simulink model "dsss"  (Simulink 7.1)
settings: Solver=ode45  StartTime=0.0  StopTime=0.80  RelTol=1e-3
libraries: simulink x264, dspbuff3 x24, dspxfrm3 x8, commsynccomp2 x5, dspsigops x4, dspobslib x4, dsparch4 x3, commutil2 x2, commseqgen2 x1, commfilt2 x1, commsink2 x1, dspspect3 x1
(part 2 of 4)

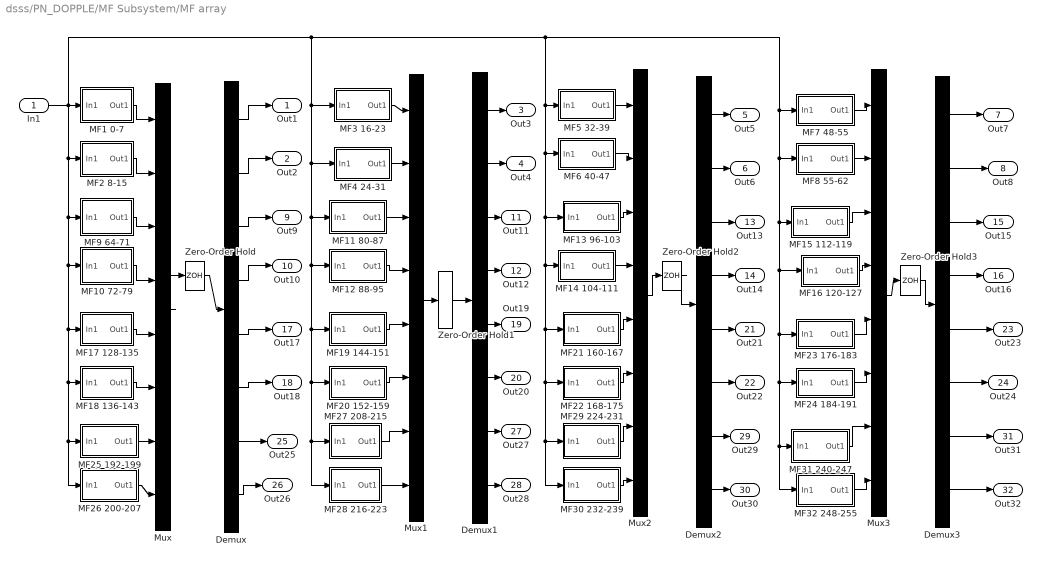
== system dsss/PN_DOPPLE/MF Subsystem/MF array ==
  In1 : Inport  OutDataType=sfix(16)  OutScaling=2^0
  Demux{,1..3} (4 alike) : Demux  Outputs=8
  MF1 0-7 : Subsystem
  MF10 72-79 : Subsystem
  MF11 80-87 : Subsystem
  MF12 88-95 : Subsystem
  MF13 96-103 : Subsystem
  MF14 104-111 : Subsystem
  MF15 112-119 : Subsystem
  MF16 120-127 : Subsystem
  MF17 128-135 : Subsystem
  MF18 136-143 : Subsystem
  MF19 144-151 : Subsystem
  MF2 8-15 : Subsystem
  MF20 152-159 : Subsystem
  MF21 160-167 : Subsystem
  MF22 168-175 : Subsystem
  MF23 176-183 : Subsystem
  MF24 184-191 : Subsystem
  MF25 192-199 : Subsystem
  MF26 200-207 : Subsystem
  MF27 208-215 : Subsystem
  MF28 216-223 : Subsystem
  MF29 224-231 : Subsystem
  MF3 16-23 : Subsystem
  MF30 232-239 : Subsystem
  MF31 240-247 : Subsystem
  MF32 248-255 : Subsystem
  MF4 24-31 : Subsystem
  MF5 32-39 : Subsystem
  MF6 40-47 : Subsystem
  MF7 48-55 : Subsystem
  MF8 55-62 : Subsystem
  MF9 64-71 : Subsystem
  Mux{,1..3} (4 alike) : Mux  Inputs=8
  Zero-Order Hold{,1..3} (4 alike) : ZeroOrderHold  SampleTime=1/255000
  Out1 : Outport  OutDataType=sfix(16)  OutScaling=2^0
  Out2 : Outport  Port=2  OutDataType=sfix(16)  OutScaling=2^0
  Out3 : Outport  Port=3  OutDataType=sfix(16)  OutScaling=2^0
  Out4 : Outport  Port=4  OutDataType=sfix(16)  OutScaling=2^0
  Out5 : Outport  Port=5  OutDataType=sfix(16)  OutScaling=2^0
  Out6 : Outport  Port=6  OutDataType=sfix(16)  OutScaling=2^0
  Out7 : Outport  Port=7  OutDataType=sfix(16)  OutScaling=2^0
  Out8 : Outport  Port=8  OutDataType=sfix(16)  OutScaling=2^0
  Out9 : Outport  Port=9  OutDataType=sfix(16)  OutScaling=2^0
  Out10 : Outport  Port=10  OutDataType=sfix(16)  OutScaling=2^0
  Out11 : Outport  Port=11  OutDataType=sfix(16)  OutScaling=2^0
  Out12 : Outport  Port=12  OutDataType=sfix(16)  OutScaling=2^0
  Out13 : Outport  Port=13  OutDataType=sfix(16)  OutScaling=2^0
  Out14 : Outport  Port=14  OutDataType=sfix(16)  OutScaling=2^0
  Out15 : Outport  Port=15  OutDataType=sfix(16)  OutScaling=2^0
  Out16 : Outport  Port=16  OutDataType=sfix(16)  OutScaling=2^0
  Out17 : Outport  Port=17  OutDataType=sfix(16)  OutScaling=2^0
  Out18 : Outport  Port=18  OutDataType=sfix(16)  OutScaling=2^0
  Out19 : Outport  Port=19  OutDataType=sfix(16)  OutScaling=2^0
  Out20 : Outport  Port=20  OutDataType=sfix(16)  OutScaling=2^0
  Out21 : Outport  Port=21  OutDataType=sfix(16)  OutScaling=2^0
  Out22 : Outport  Port=22  OutDataType=sfix(16)  OutScaling=2^0
  Out23 : Outport  Port=23  OutDataType=sfix(16)  OutScaling=2^0
  Out24 : Outport  Port=24  OutDataType=sfix(16)  OutScaling=2^0
  Out25 : Outport  Port=25  OutDataType=sfix(16)  OutScaling=2^0
  Out26 : Outport  Port=26  OutDataType=sfix(16)  OutScaling=2^0
  Out27 : Outport  Port=27  OutDataType=sfix(16)  OutScaling=2^0
  Out28 : Outport  Port=28  OutDataType=sfix(16)  OutScaling=2^0
  Out29 : Outport  Port=29  OutDataType=sfix(16)  OutScaling=2^0
  Out30 : Outport  Port=30  OutDataType=sfix(16)  OutScaling=2^0
  Out31 : Outport  Port=31  OutDataType=sfix(16)  OutScaling=2^0
  Out32 : Outport  Port=32  OutDataType=sfix(16)  OutScaling=2^0
  wires:
  Zero-Order Hold3/1 -> Demux3/1
  Mux3/1 -> Zero-Order Hold3/1
  Zero-Order Hold2/1 -> Demux2/1
  Mux2/1 -> Zero-Order Hold2/1
  Zero-Order Hold1/1 -> Demux1/1
  Mux1/1 -> Zero-Order Hold1/1
  Zero-Order Hold/1 -> Demux/1
  Mux/1 -> Zero-Order Hold/1
  In1/1 -> MF1 0-7/1(In1), MF3 16-23/1(In1), MF11 80-87/1(In1), MF19 144-151/1(In1), MF20 152-159/1(In1), MF27 208-215/1(In1), MF28 216-223/1(In1), MF12 88-95/1(In1), MF4 24-31/1(In1), MF5 32-39/1(In1), MF13 96-103/1(In1), MF21 160-167/1(In1), MF22 168-175/1(In1), MF29 224-231/1(In1), MF30 232-239/1(In1), MF14 104-111/1(In1), MF6 40-47/1(In1), MF7 48-55/1(In1), MF23 176-183/1(In1), MF24 184-191/1(In1), MF31 240-247/1(In1), MF32 248-255/1(In1), MF16 120-127/1(In1), MF15 112-119/1(In1), MF8 55-62/1(In1), MF9 64-71/1(In1), MF17 128-135/1(In1), MF18 136-143/1(In1), MF25 192-199/1(In1), MF26 200-207/1(In1), MF10 72-79/1(In1), MF2 8-15/1(In1)
  MF1 0-7/1(Out1) -> Mux/1
  MF2 8-15/1(Out1) -> Mux/2
  MF9 64-71/1(Out1) -> Mux/3
  MF10 72-79/1(Out1) -> Mux/4
  MF17 128-135/1(Out1) -> Mux/5
  MF18 136-143/1(Out1) -> Mux/6
  MF25 192-199/1(Out1) -> Mux/7
  MF26 200-207/1(Out1) -> Mux/8
  Demux/1 -> Out1/1
  Demux/2 -> Out2/1
  Demux/3 -> Out9/1
  Demux/4 -> Out10/1
  Demux/5 -> Out17/1
  Demux/6 -> Out18/1
  Demux/7 -> Out25/1
  Demux/8 -> Out26/1
  MF3 16-23/1(Out1) -> Mux1/1
  MF4 24-31/1(Out1) -> Mux1/2
  MF11 80-87/1(Out1) -> Mux1/3
  MF12 88-95/1(Out1) -> Mux1/4
  MF19 144-151/1(Out1) -> Mux1/5
  MF20 152-159/1(Out1) -> Mux1/6
  MF27 208-215/1(Out1) -> Mux1/7
  MF28 216-223/1(Out1) -> Mux1/8
  Demux1/1 -> Out3/1
  Demux1/2 -> Out4/1
  Demux1/3 -> Out11/1
  Demux1/4 -> Out12/1
  Demux1/5 -> Out19/1
  Demux1/6 -> Out20/1
  Demux1/7 -> Out27/1
  Demux1/8 -> Out28/1
  MF5 32-39/1(Out1) -> Mux2/1
  MF6 40-47/1(Out1) -> Mux2/2
  MF13 96-103/1(Out1) -> Mux2/3
  MF14 104-111/1(Out1) -> Mux2/4
  MF21 160-167/1(Out1) -> Mux2/5
  MF22 168-175/1(Out1) -> Mux2/6
  MF29 224-231/1(Out1) -> Mux2/7
  MF30 232-239/1(Out1) -> Mux2/8
  Demux2/1 -> Out5/1
  Demux2/2 -> Out6/1
  Demux2/3 -> Out13/1
  Demux2/4 -> Out14/1
  Demux2/5 -> Out21/1
  Demux2/6 -> Out22/1
  Demux2/7 -> Out29/1
  Demux2/8 -> Out30/1
  MF7 48-55/1(Out1) -> Mux3/1
  MF8 55-62/1(Out1) -> Mux3/2
  MF15 112-119/1(Out1) -> Mux3/3
  MF16 120-127/1(Out1) -> Mux3/4
  MF23 176-183/1(Out1) -> Mux3/5
  MF24 184-191/1(Out1) -> Mux3/6
  MF31 240-247/1(Out1) -> Mux3/7
  MF32 248-255/1(Out1) -> Mux3/8
  Demux3/1 -> Out7/1
  Demux3/2 -> Out8/1
  Demux3/3 -> Out15/1
  Demux3/4 -> Out16/1
  Demux3/5 -> Out23/1
  Demux3/6 -> Out24/1
  Demux3/7 -> Out31/1
  Demux3/8 -> Out32/1

== system dsss/PN_DOPPLE/FFT compensate/Subsystem/Subsystem ==
  In1 : Inport  OutDataType=sfix(16)  OutScaling=2^0
  Constant : Constant  OutDataType=sfix(16)  OutScaling=2^0
  Constant1 : Constant  Value=0  OutDataType=sfix(16)  OutScaling=2^0
  Constant2 : Constant  Value=0  OutDataType=sfix(16)  OutScaling=2^0
  Product : Product  OutDataType=sfix(16)  OutScaling=2^0  RndMeth=Zero
  Switch : Switch  Threshold=65
  Out1 : Outport  OutDataType=sfix(16)  OutScaling=2^0
  wires:
  Constant/1 -> Switch/1
  Constant1/1 -> Switch/3
  Switch/1 -> Product/1
  Constant2/1 -> Product/2
  In1/1 -> Switch/2
  Product/1 -> Out1/1

== system dsss/PN_DOPPLE/FFT compensate/Subsystem/Subsystem1 ==
  In1 : Inport  OutDataType=sfix(16)  OutScaling=2^0
  Constant : Constant  OutDataType=sfix(16)  OutScaling=2^0
  Constant1 : Constant  Value=0  OutDataType=sfix(16)  OutScaling=2^0
  Constant2 : Constant  Value=10  OutDataType=sfix(16)  OutScaling=2^0
  Product : Product  OutDataType=sfix(16)  OutScaling=2^0  RndMeth=Zero
  Switch : Switch  Threshold=65
  Out1 : Outport  OutDataType=sfix(16)  OutScaling=2^0
  wires:
  Product/1 -> Out1/1
  In1/1 -> Switch/2
  Constant2/1 -> Product/2
  Switch/1 -> Product/1
  Constant1/1 -> Switch/3
  Constant/1 -> Switch/1

== system dsss/PN_DOPPLE/FFT compensate/Subsystem/Subsystem10 ==
  In1 : Inport  OutDataType=sfix(16)  OutScaling=2^0
  Constant : Constant  OutDataType=sfix(16)  OutScaling=2^0
  Constant1 : Constant  Value=0  OutDataType=sfix(16)  OutScaling=2^0
  Constant2 : Constant  Value=100  OutDataType=sfix(16)  OutScaling=2^0
  Product : Product  OutDataType=sfix(16)  OutScaling=2^0  RndMeth=Zero
  Switch : Switch  Threshold=65
  Out1 : Outport  OutDataType=sfix(16)  OutScaling=2^0
  wires:
  Constant/1 -> Switch/1
  Constant1/1 -> Switch/3
  Switch/1 -> Product/1
  Constant2/1 -> Product/2
  In1/1 -> Switch/2
  Product/1 -> Out1/1

== system dsss/PN_DOPPLE/FFT compensate/Subsystem/Subsystem11 ==
  In1 : Inport  OutDataType=sfix(16)  OutScaling=2^0
  Constant : Constant  OutDataType=sfix(16)  OutScaling=2^0
  Constant1 : Constant  Value=0  OutDataType=sfix(16)  OutScaling=2^0
  Constant2 : Constant  Value=110  OutDataType=sfix(16)  OutScaling=2^0
  Product : Product  OutDataType=sfix(16)  OutScaling=2^0  RndMeth=Zero
  Switch : Switch  Threshold=65
  Out1 : Outport  OutDataType=sfix(16)  OutScaling=2^0
  wires:
  Product/1 -> Out1/1
  In1/1 -> Switch/2
  Constant2/1 -> Product/2
  Switch/1 -> Product/1
  Constant1/1 -> Switch/3
  Constant/1 -> Switch/1

== system dsss/PN_DOPPLE/FFT compensate/Subsystem/Subsystem12 ==
  In1 : Inport  OutDataType=sfix(16)  OutScaling=2^0
  Constant : Constant  OutDataType=sfix(16)  OutScaling=2^0
  Constant1 : Constant  Value=0  OutDataType=sfix(16)  OutScaling=2^0
  Constant2 : Constant  Value=120  OutDataType=sfix(16)  OutScaling=2^0
  Product : Product  OutDataType=sfix(16)  OutScaling=2^0  RndMeth=Zero
  Switch : Switch  Threshold=65
  Out1 : Outport  OutDataType=sfix(16)  OutScaling=2^0
  wires:
  Constant/1 -> Switch/1
  Constant1/1 -> Switch/3
  Switch/1 -> Product/1
  Constant2/1 -> Product/2
  In1/1 -> Switch/2
  Product/1 -> Out1/1

== system dsss/PN_DOPPLE/FFT compensate/Subsystem/Subsystem13 ==
  In1 : Inport  OutDataType=sfix(16)  OutScaling=2^0
  Constant : Constant  OutDataType=sfix(16)  OutScaling=2^0
  Constant1 : Constant  Value=0  OutDataType=sfix(16)  OutScaling=2^0
  Constant2 : Constant  Value=130  OutDataType=sfix(16)  OutScaling=2^0
  Product : Product  OutDataType=sfix(16)  OutScaling=2^0  RndMeth=Zero
  Switch : Switch  Threshold=65
  Out1 : Outport  OutDataType=sfix(16)  OutScaling=2^0
  wires:
  Product/1 -> Out1/1
  In1/1 -> Switch/2
  Constant2/1 -> Product/2
  Switch/1 -> Product/1
  Constant1/1 -> Switch/3
  Constant/1 -> Switch/1

== system dsss/PN_DOPPLE/FFT compensate/Subsystem/Subsystem14 ==
  In1 : Inport  OutDataType=sfix(16)  OutScaling=2^0
  Constant : Constant  OutDataType=sfix(16)  OutScaling=2^0
  Constant1 : Constant  Value=0  OutDataType=sfix(16)  OutScaling=2^0
  Constant2 : Constant  Value=140  OutDataType=sfix(16)  OutScaling=2^0
  Product : Product  OutDataType=sfix(16)  OutScaling=2^0  RndMeth=Zero
  Switch : Switch  Threshold=65
  Out1 : Outport  OutDataType=sfix(16)  OutScaling=2^0
  wires:
  Constant/1 -> Switch/1
  Constant1/1 -> Switch/3
  Switch/1 -> Product/1
  Constant2/1 -> Product/2
  In1/1 -> Switch/2
  Product/1 -> Out1/1

== system dsss/PN_DOPPLE/FFT compensate/Subsystem/Subsystem15 ==
  In1 : Inport  OutDataType=sfix(16)  OutScaling=2^0
  Constant : Constant  OutDataType=sfix(16)  OutScaling=2^0
  Constant1 : Constant  Value=0  OutDataType=sfix(16)  OutScaling=2^0
  Constant2 : Constant  Value=150  OutDataType=sfix(16)  OutScaling=2^0
  Product : Product  OutDataType=sfix(16)  OutScaling=2^0  RndMeth=Zero
  Switch : Switch  Threshold=65
  Out1 : Outport  OutDataType=sfix(16)  OutScaling=2^0
  wires:
  Product/1 -> Out1/1
  In1/1 -> Switch/2
  Constant2/1 -> Product/2
  Switch/1 -> Product/1
  Constant1/1 -> Switch/3
  Constant/1 -> Switch/1

== system dsss/PN_DOPPLE/FFT compensate/Subsystem/Subsystem2 ==
  In1 : Inport  OutDataType=sfix(16)  OutScaling=2^0
  Constant : Constant  OutDataType=sfix(16)  OutScaling=2^0
  Constant1 : Constant  Value=0  OutDataType=sfix(16)  OutScaling=2^0
  Constant2 : Constant  Value=20  OutDataType=sfix(16)  OutScaling=2^0
  Product : Product  OutDataType=sfix(16)  OutScaling=2^0  RndMeth=Zero
  Switch : Switch  Threshold=65
  Out1 : Outport  OutDataType=sfix(16)  OutScaling=2^0
  wires:
  Constant/1 -> Switch/1
  Constant1/1 -> Switch/3
  Switch/1 -> Product/1
  Constant2/1 -> Product/2
  In1/1 -> Switch/2
  Product/1 -> Out1/1

== system dsss/PN_DOPPLE/FFT compensate/Subsystem/Subsystem3 ==
  In1 : Inport  OutDataType=sfix(16)  OutScaling=2^0
  Constant : Constant  OutDataType=sfix(16)  OutScaling=2^0
  Constant1 : Constant  Value=0  OutDataType=sfix(16)  OutScaling=2^0
  Constant2 : Constant  Value=30  OutDataType=sfix(16)  OutScaling=2^0
  Product : Product  OutDataType=sfix(16)  OutScaling=2^0  RndMeth=Zero
  Switch : Switch  Threshold=65
  Out1 : Outport  OutDataType=sfix(16)  OutScaling=2^0
  wires:
  Product/1 -> Out1/1
  In1/1 -> Switch/2
  Constant2/1 -> Product/2
  Switch/1 -> Product/1
  Constant1/1 -> Switch/3
  Constant/1 -> Switch/1

== system dsss/PN_DOPPLE/FFT compensate/Subsystem/Subsystem4 ==
  In1 : Inport  OutDataType=sfix(16)  OutScaling=2^0
  Constant : Constant  OutDataType=sfix(16)  OutScaling=2^0
  Constant1 : Constant  Value=0  OutDataType=sfix(16)  OutScaling=2^0
  Constant2 : Constant  Value=40  OutDataType=sfix(16)  OutScaling=2^0
  Product : Product  OutDataType=sfix(16)  OutScaling=2^0  RndMeth=Zero
  Switch : Switch  Threshold=65
  Out1 : Outport  OutDataType=sfix(16)  OutScaling=2^0
  wires:
  Constant/1 -> Switch/1
  Constant1/1 -> Switch/3
  Switch/1 -> Product/1
  Constant2/1 -> Product/2
  In1/1 -> Switch/2
  Product/1 -> Out1/1

== system dsss/PN_DOPPLE/FFT compensate/Subsystem/Subsystem5 ==
  In1 : Inport  OutDataType=sfix(16)  OutScaling=2^0
  Constant : Constant  OutDataType=sfix(16)  OutScaling=2^0
  Constant1 : Constant  Value=0  OutDataType=sfix(16)  OutScaling=2^0
  Constant2 : Constant  Value=50  OutDataType=sfix(16)  OutScaling=2^0
  Product : Product  OutDataType=sfix(16)  OutScaling=2^0  RndMeth=Zero
  Switch : Switch  Threshold=65
  Out1 : Outport  OutDataType=sfix(16)  OutScaling=2^0
  wires:
  Product/1 -> Out1/1
  In1/1 -> Switch/2
  Constant2/1 -> Product/2
  Switch/1 -> Product/1
  Constant1/1 -> Switch/3
  Constant/1 -> Switch/1

== system dsss/PN_DOPPLE/FFT compensate/Subsystem/Subsystem6 ==
  In1 : Inport  OutDataType=sfix(16)  OutScaling=2^0
  Constant : Constant  OutDataType=sfix(16)  OutScaling=2^0
  Constant1 : Constant  Value=0  OutDataType=sfix(16)  OutScaling=2^0
  Constant2 : Constant  Value=60  OutDataType=sfix(16)  OutScaling=2^0
  Product : Product  OutDataType=sfix(16)  OutScaling=2^0  RndMeth=Zero
  Switch : Switch  Threshold=65
  Out1 : Outport  OutDataType=sfix(16)  OutScaling=2^0
  wires:
  Constant/1 -> Switch/1
  Constant1/1 -> Switch/3
  Switch/1 -> Product/1
  Constant2/1 -> Product/2
  In1/1 -> Switch/2
  Product/1 -> Out1/1

== system dsss/PN_DOPPLE/FFT compensate/Subsystem/Subsystem7 ==
  In1 : Inport  OutDataType=sfix(16)  OutScaling=2^0
  Constant : Constant  OutDataType=sfix(16)  OutScaling=2^0
  Constant1 : Constant  Value=0  OutDataType=sfix(16)  OutScaling=2^0
  Constant2 : Constant  Value=70  OutDataType=sfix(16)  OutScaling=2^0
  Product : Product  OutDataType=sfix(16)  OutScaling=2^0  RndMeth=Zero
  Switch : Switch  Threshold=65
  Out1 : Outport  OutDataType=sfix(16)  OutScaling=2^0
  wires:
  Product/1 -> Out1/1
  In1/1 -> Switch/2
  Constant2/1 -> Product/2
  Switch/1 -> Product/1
  Constant1/1 -> Switch/3
  Constant/1 -> Switch/1

== system dsss/PN_DOPPLE/FFT compensate/Subsystem/Subsystem8 ==
  In1 : Inport  OutDataType=sfix(16)  OutScaling=2^0
  Constant : Constant  OutDataType=sfix(16)  OutScaling=2^0
  Constant1 : Constant  Value=0  OutDataType=sfix(16)  OutScaling=2^0
  Constant2 : Constant  Value=80  OutDataType=sfix(16)  OutScaling=2^0
  Product : Product  OutDataType=sfix(16)  OutScaling=2^0  RndMeth=Zero
  Switch : Switch  Threshold=65
  Out1 : Outport  OutDataType=sfix(16)  OutScaling=2^0
  wires:
  Constant/1 -> Switch/1
  Constant1/1 -> Switch/3
  Switch/1 -> Product/1
  Constant2/1 -> Product/2
  In1/1 -> Switch/2
  Product/1 -> Out1/1

== system dsss/PN_DOPPLE/FFT compensate/Subsystem/Subsystem9 ==
  In1 : Inport  OutDataType=sfix(16)  OutScaling=2^0
  Constant : Constant  OutDataType=sfix(16)  OutScaling=2^0
  Constant1 : Constant  Value=0  OutDataType=sfix(16)  OutScaling=2^0
  Constant2 : Constant  Value=90  OutDataType=sfix(16)  OutScaling=2^0
  Product : Product  OutDataType=sfix(16)  OutScaling=2^0  RndMeth=Zero
  Switch : Switch  Threshold=65
  Out1 : Outport  OutDataType=sfix(16)  OutScaling=2^0
  wires:
  Product/1 -> Out1/1
  In1/1 -> Switch/2
  Constant2/1 -> Product/2
  Switch/1 -> Product/1
  Constant1/1 -> Switch/3
  Constant/1 -> Switch/1

== system dsss/PN_DOPPLE/Local PN/local PN sequence Include Track/Clock ==
  In2 : Inport  Orientation=left  OutDataType=sfix(16)  OutScaling=2^0
  Constant : Constant  Orientation=left  OutDataType=sfix(16)  OutScaling=2^0
  Constant1 : Constant  Orientation=left  Value=0  OutDataType=sfix(16)  OutScaling=2^0
  Continuous-Time VCO : commsynccomp2/Continuous-Time VCO  Orientation=left  SystemSampleTime=-1  Ac=1  Fc=255000  Kc=0.15  Ph=-pi/2
  Switch : Switch  Orientation=left
  Out1 : Outport  Orientation=left  OutDataType=sfix(16)  OutScaling=2^0
  wires:
  Constant1/1 -> Switch/3
  Constant/1 -> Switch/1
  Continuous-Time VCO/1 -> Switch/2
  Switch/1 -> Out1/1
  In2/1 -> Continuous-Time VCO/1

== system dsss/PN_DOPPLE/Local PN/local PN sequence Include Track/Local System ==
  In1 : Inport  OutDataType=sfix(16)  OutScaling=2^0
  Data Type Conversion : DataTypeConversion  OutDataTypeMode=double  OutDataType=sfix(16)  OutScaling=2^0  OutDataTypeStr=double
  Zero-Order Hold3 : ZeroOrderHold  SampleTime=1/255e3
  "[1 0 0 1 1 1 0 1]PN" : Subsystem  TreatAsAtomicUnit=on
  "[1 0 0 1 1 1 0 1]" : Outport  OutDataType=sfix(16)  OutScaling=2^0
  wires:
  In1/1 -> "[1 0 0 1 1 1 0 1]PN"/Trigger, "[1 0 0 1 1 1 0 1]PN"/1(In1)
  "[1 0 0 1 1 1 0 1]PN"/1(Out1) -> Data Type Conversion/1
  Zero-Order Hold3/1 -> "[1 0 0 1 1 1 0 1]"/1
  Data Type Conversion/1 -> Zero-Order Hold3/1

== system dsss/PN_DOPPLE/Local PN/logic control/Triggered Subsystem ==
  Trigger : TriggerPort
  Constant : Constant  OutDataType=sfix(16)  OutScaling=2^0
  Logical Operator : Logic  Operator=XOR  AllPortsSameDT=off  OutDataTypeMode=boolean  OutDataTypeStr=boolean
  Scope : Scope
      settings: SaveName=ScopeData2
  Unit Delay : UnitDelay  Orientation=left  SampleTime=-1
  Out2 : Outport  OutDataType=sfix(16)  OutScaling=2^0
  wires:
  Constant/1 -> Logical Operator/1
  Logical Operator/1 -> Scope/1, Out2/1, Unit Delay/1
  Unit Delay/1 -> Logical Operator/2

== system dsss/PN_DOPPLE/Local PN/threshold deside stop and start/Triggered Subsystem ==
  Trigger : TriggerPort
  Constant1 : Constant  OutDataType=sfix(16)  OutScaling=2^0
  Logical Operator : Logic  Operator=XOR  AllPortsSameDT=off  OutDataTypeMode=boolean  OutDataTypeStr=boolean
  Unit Delay : UnitDelay  Orientation=left  SampleTime=-1
  Out1 : Outport  OutDataType=sfix(16)  OutScaling=2^0
  wires:
  Unit Delay/1 -> Logical Operator/2
  Logical Operator/1 -> Out1/1, Unit Delay/1
  Constant1/1 -> Logical Operator/1

== system dsss/PN_DOPPLE/MF Subsystem/MF array/MF1 0-7 ==
  In1 : Inport  OutDataType=sfix(16)  OutScaling=2^0
  Add : Sum  Inputs=++++++++  OutDataType=sfix(16)  OutScaling=2^-10
  Subsystem : Subsystem
  Out1 : Outport  OutDataType=sfix(16)  OutScaling=2^0
  wires:
  Add/1 -> Out1/1
  In1/1 -> Subsystem/1(In1)
  Subsystem/1(Out1) -> Add/1
  Subsystem/2(Out2) -> Add/2
  Subsystem/3(Out3) -> Add/3
  Subsystem/4(Out4) -> Add/4
  Subsystem/5(Out5) -> Add/5
  Subsystem/6(Out6) -> Add/6
  Subsystem/7(Out7) -> Add/7
  Subsystem/8(Out8) -> Add/8

== system dsss/PN_DOPPLE/MF Subsystem/MF array/MF10 72-79 ==
  In1 : Inport  OutDataType=sfix(16)  OutScaling=2^0
  Add : Sum  Inputs=++++++++  OutDataType=sfix(16)  OutScaling=2^-10
  Subsystem : Subsystem
  Out1 : Outport  OutDataType=sfix(16)  OutScaling=2^0
  wires:
  Subsystem/8(Out8) -> Add/8
  Subsystem/7(Out7) -> Add/7
  Subsystem/6(Out6) -> Add/6
  Subsystem/5(Out5) -> Add/5
  Subsystem/4(Out4) -> Add/4
  Subsystem/3(Out3) -> Add/3
  Subsystem/2(Out2) -> Add/2
  Subsystem/1(Out1) -> Add/1
  In1/1 -> Subsystem/1(In1)
  Add/1 -> Out1/1

== system dsss/PN_DOPPLE/MF Subsystem/MF array/MF11 80-87 ==
  In1 : Inport  OutDataType=sfix(16)  OutScaling=2^0
  Add : Sum  Inputs=++++++++  OutDataType=sfix(16)  OutScaling=2^-10
  Subsystem : Subsystem
  Out1 : Outport  OutDataType=sfix(16)  OutScaling=2^0
  wires:
  In1/1 -> Subsystem/1(In1)
  Add/1 -> Out1/1
  Subsystem/1(Out3) -> Add/1
  Subsystem/2(Out4) -> Add/2
  Subsystem/3(Out7) -> Add/3
  Subsystem/4(Out8) -> Add/4
  Subsystem/5(Out9) -> Add/5
  Subsystem/6(Out11) -> Add/6
  Subsystem/7(Out14) -> Add/7
  Subsystem/8(Out15) -> Add/8

== system dsss/PN_DOPPLE/MF Subsystem/MF array/MF12 88-95 ==
  In1 : Inport  OutDataType=sfix(16)  OutScaling=2^0
  Add : Sum  Inputs=++++++++  OutDataType=sfix(16)  OutScaling=2^-10
  Subsystem : Subsystem
  Out1 : Outport  OutDataType=sfix(16)  OutScaling=2^0
  wires:
  Add/1 -> Out1/1
  In1/1 -> Subsystem/1(In1)
  Subsystem/1(Out1) -> Add/1
  Subsystem/2(Out5) -> Add/2
  Subsystem/3(Out10) -> Add/3
  Subsystem/4(Out12) -> Add/4
  Subsystem/5(Out13) -> Add/5
  Subsystem/6(Out16) -> Add/6
  Subsystem/7(Out17) -> Add/7
  Subsystem/8(Out18) -> Add/8

== system dsss/PN_DOPPLE/MF Subsystem/MF array/MF13 96-103 ==
  In1 : Inport  OutDataType=sfix(16)  OutScaling=2^0
  Add : Sum  Inputs=++++++++  OutDataType=sfix(16)  OutScaling=2^-10
  Subsystem : Subsystem
  Out1 : Outport  OutDataType=sfix(16)  OutScaling=2^0
  wires:
  Add/1 -> Out1/1
  In1/1 -> Subsystem/1(In1)
  Subsystem/1(Out3) -> Add/1
  Subsystem/2(Out4) -> Add/2
  Subsystem/3(Out7) -> Add/3
  Subsystem/4(Out8) -> Add/4
  Subsystem/5(Out9) -> Add/5
  Subsystem/6(Out11) -> Add/6
  Subsystem/7(Out14) -> Add/7
  Subsystem/8(Out15) -> Add/8

== system dsss/PN_DOPPLE/MF Subsystem/MF array/MF14 104-111 ==
  In1 : Inport  OutDataType=sfix(16)  OutScaling=2^0
  Add : Sum  Inputs=++++++++  OutDataType=sfix(16)  OutScaling=2^-10
  Subsystem : Subsystem
  Out1 : Outport  OutDataType=sfix(16)  OutScaling=2^0
  wires:
  In1/1 -> Subsystem/1(In1)
  Add/1 -> Out1/1
  Subsystem/1(Out1) -> Add/1
  Subsystem/2(Out5) -> Add/2
  Subsystem/3(Out10) -> Add/3
  Subsystem/4(Out12) -> Add/4
  Subsystem/5(Out13) -> Add/5
  Subsystem/6(Out16) -> Add/6
  Subsystem/7(Out17) -> Add/7
  Subsystem/8(Out18) -> Add/8

== system dsss/PN_DOPPLE/MF Subsystem/MF array/MF15 112-119 ==
  In1 : Inport  OutDataType=sfix(16)  OutScaling=2^0
  Add : Sum  Inputs=++++++++  OutDataType=sfix(16)  OutScaling=2^-10
  Subsystem : Subsystem
  Out1 : Outport  OutDataType=sfix(16)  OutScaling=2^0
  wires:
  In1/1 -> Subsystem/1(In1)
  Add/1 -> Out1/1
  Subsystem/1(Out3) -> Add/1
  Subsystem/2(Out4) -> Add/2
  Subsystem/3(Out7) -> Add/3
  Subsystem/4(Out8) -> Add/4
  Subsystem/5(Out9) -> Add/5
  Subsystem/6(Out11) -> Add/6
  Subsystem/7(Out14) -> Add/7
  Subsystem/8(Out15) -> Add/8

== system dsss/PN_DOPPLE/MF Subsystem/MF array/MF16 120-127 ==
  In1 : Inport  OutDataType=sfix(16)  OutScaling=2^0
  Add : Sum  Inputs=++++++++  OutDataType=sfix(16)  OutScaling=2^-10
  Subsystem : Subsystem
  Out1 : Outport  OutDataType=sfix(16)  OutScaling=2^0
  wires:
  Add/1 -> Out1/1
  In1/1 -> Subsystem/1(In1)
  Subsystem/1(Out1) -> Add/1
  Subsystem/2(Out5) -> Add/2
  Subsystem/3(Out10) -> Add/3
  Subsystem/4(Out12) -> Add/4
  Subsystem/5(Out13) -> Add/5
  Subsystem/6(Out16) -> Add/6
  Subsystem/7(Out17) -> Add/7
  Subsystem/8(Out18) -> Add/8

== system dsss/PN_DOPPLE/MF Subsystem/MF array/MF17 128-135 ==
  In1 : Inport  OutDataType=sfix(16)  OutScaling=2^0
  Add : Sum  Inputs=++++++++  OutDataType=sfix(16)  OutScaling=2^-10
  Subsystem : Subsystem
  Out1 : Outport  OutDataType=sfix(16)  OutScaling=2^0
  wires:
  In1/1 -> Subsystem/1(In1)
  Add/1 -> Out1/1
  Subsystem/1(Out3) -> Add/1
  Subsystem/2(Out4) -> Add/2
  Subsystem/3(Out7) -> Add/3
  Subsystem/4(Out8) -> Add/4
  Subsystem/5(Out9) -> Add/5
  Subsystem/6(Out11) -> Add/6
  Subsystem/7(Out14) -> Add/7
  Subsystem/8(Out15) -> Add/8

== system dsss/PN_DOPPLE/MF Subsystem/MF array/MF18 136-143 ==
  In1 : Inport  OutDataType=sfix(16)  OutScaling=2^0
  Add : Sum  Inputs=++++++++  OutDataType=sfix(16)  OutScaling=2^-10
  Subsystem : Subsystem
  Out1 : Outport  OutDataType=sfix(16)  OutScaling=2^0
  wires:
  Add/1 -> Out1/1
  In1/1 -> Subsystem/1(In1)
  Subsystem/1(Out1) -> Add/1
  Subsystem/2(Out5) -> Add/2
  Subsystem/3(Out10) -> Add/3
  Subsystem/4(Out12) -> Add/4
  Subsystem/5(Out13) -> Add/5
  Subsystem/6(Out16) -> Add/6
  Subsystem/7(Out17) -> Add/7
  Subsystem/8(Out18) -> Add/8

== system dsss/PN_DOPPLE/MF Subsystem/MF array/MF19 144-151 ==
  In1 : Inport  OutDataType=sfix(16)  OutScaling=2^0
  Add : Sum  Inputs=++++++++  OutDataType=sfix(16)  OutScaling=2^-10
  Subsystem : Subsystem
  Out1 : Outport  OutDataType=sfix(16)  OutScaling=2^0
  wires:
  Add/1 -> Out1/1
  In1/1 -> Subsystem/1(In1)
  Subsystem/1(Out3) -> Add/1
  Subsystem/2(Out4) -> Add/2
  Subsystem/3(Out7) -> Add/3
  Subsystem/4(Out8) -> Add/4
  Subsystem/5(Out9) -> Add/5
  Subsystem/6(Out11) -> Add/6
  Subsystem/7(Out14) -> Add/7
  Subsystem/8(Out15) -> Add/8

== system dsss/PN_DOPPLE/MF Subsystem/MF array/MF2 8-15 ==
  In1 : Inport  OutDataType=sfix(16)  OutScaling=2^0
  Add : Sum  Inputs=++++++++  OutDataType=sfix(16)  OutScaling=2^-10
  Subsystem : Subsystem
  Out1 : Outport  OutDataType=sfix(16)  OutScaling=2^0
  wires:
  Subsystem/8(Out8) -> Add/8
  Subsystem/7(Out7) -> Add/7
  Subsystem/6(Out6) -> Add/6
  Subsystem/5(Out5) -> Add/5
  Subsystem/4(Out4) -> Add/4
  Subsystem/3(Out3) -> Add/3
  Subsystem/2(Out2) -> Add/2
  Subsystem/1(Out1) -> Add/1
  In1/1 -> Subsystem/1(In1)
  Add/1 -> Out1/1

== system dsss/PN_DOPPLE/MF Subsystem/MF array/MF20 152-159 ==
  In1 : Inport  OutDataType=sfix(16)  OutScaling=2^0
  Add : Sum  Inputs=++++++++  OutDataType=sfix(16)  OutScaling=2^-10
  Subsystem : Subsystem
  Out1 : Outport  OutDataType=sfix(16)  OutScaling=2^0
  wires:
  In1/1 -> Subsystem/1(In1)
  Add/1 -> Out1/1
  Subsystem/1(Out1) -> Add/1
  Subsystem/2(Out5) -> Add/2
  Subsystem/3(Out10) -> Add/3
  Subsystem/4(Out12) -> Add/4
  Subsystem/5(Out13) -> Add/5
  Subsystem/6(Out16) -> Add/6
  Subsystem/7(Out17) -> Add/7
  Subsystem/8(Out18) -> Add/8

== system dsss/PN_DOPPLE/MF Subsystem/MF array/MF21 160-167 ==
  In1 : Inport  OutDataType=sfix(16)  OutScaling=2^0
  Add : Sum  Inputs=++++++++  OutDataType=sfix(16)  OutScaling=2^-10
  Subsystem : Subsystem
  Out1 : Outport  OutDataType=sfix(16)  OutScaling=2^0
  wires:
  In1/1 -> Subsystem/1(In1)
  Add/1 -> Out1/1
  Subsystem/1(Out3) -> Add/1
  Subsystem/2(Out4) -> Add/2
  Subsystem/3(Out7) -> Add/3
  Subsystem/4(Out8) -> Add/4
  Subsystem/5(Out9) -> Add/5
  Subsystem/6(Out11) -> Add/6
  Subsystem/7(Out14) -> Add/7
  Subsystem/8(Out15) -> Add/8

== system dsss/PN_DOPPLE/MF Subsystem/MF array/MF22 168-175 ==
  In1 : Inport  OutDataType=sfix(16)  OutScaling=2^0
  Add : Sum  Inputs=++++++++  OutDataType=sfix(16)  OutScaling=2^-10
  Subsystem : Subsystem
  Out1 : Outport  OutDataType=sfix(16)  OutScaling=2^0
  wires:
  Add/1 -> Out1/1
  In1/1 -> Subsystem/1(In1)
  Subsystem/1(Out1) -> Add/1
  Subsystem/2(Out5) -> Add/2
  Subsystem/3(Out10) -> Add/3
  Subsystem/4(Out12) -> Add/4
  Subsystem/5(Out13) -> Add/5
  Subsystem/6(Out16) -> Add/6
  Subsystem/7(Out17) -> Add/7
  Subsystem/8(Out18) -> Add/8

== system dsss/PN_DOPPLE/MF Subsystem/MF array/MF23 176-183 ==
  In1 : Inport  OutDataType=sfix(16)  OutScaling=2^0
  Add : Sum  Inputs=++++++++  OutDataType=sfix(16)  OutScaling=2^-10
  Subsystem : Subsystem
  Out1 : Outport  OutDataType=sfix(16)  OutScaling=2^0
  wires:
  Add/1 -> Out1/1
  In1/1 -> Subsystem/1(In1)
  Subsystem/1(Out3) -> Add/1
  Subsystem/2(Out4) -> Add/2
  Subsystem/3(Out7) -> Add/3
  Subsystem/4(Out8) -> Add/4
  Subsystem/5(Out9) -> Add/5
  Subsystem/6(Out11) -> Add/6
  Subsystem/7(Out14) -> Add/7
  Subsystem/8(Out15) -> Add/8

== system dsss/PN_DOPPLE/MF Subsystem/MF array/MF24 184-191 ==
  In1 : Inport  OutDataType=sfix(16)  OutScaling=2^0
  Add : Sum  Inputs=++++++++  OutDataType=sfix(16)  OutScaling=2^-10
  Subsystem : Subsystem
  Out1 : Outport  OutDataType=sfix(16)  OutScaling=2^0
  wires:
  In1/1 -> Subsystem/1(In1)
  Add/1 -> Out1/1
  Subsystem/1(Out1) -> Add/1
  Subsystem/2(Out5) -> Add/2
  Subsystem/3(Out10) -> Add/3
  Subsystem/4(Out12) -> Add/4
  Subsystem/5(Out13) -> Add/5
  Subsystem/6(Out16) -> Add/6
  Subsystem/7(Out17) -> Add/7
  Subsystem/8(Out18) -> Add/8

== system dsss/PN_DOPPLE/MF Subsystem/MF array/MF25 192-199 ==
  In1 : Inport  OutDataType=sfix(16)  OutScaling=2^0
  Add : Sum  Inputs=++++++++  OutDataType=sfix(16)  OutScaling=2^-10
  Subsystem : Subsystem
  Out1 : Outport  OutDataType=sfix(16)  OutScaling=2^0
  wires:
  In1/1 -> Subsystem/1(In1)
  Add/1 -> Out1/1
  Subsystem/1(Out3) -> Add/1
  Subsystem/2(Out4) -> Add/2
  Subsystem/3(Out7) -> Add/3
  Subsystem/4(Out8) -> Add/4
  Subsystem/5(Out9) -> Add/5
  Subsystem/6(Out11) -> Add/6
  Subsystem/7(Out14) -> Add/7
  Subsystem/8(Out15) -> Add/8

== system dsss/PN_DOPPLE/MF Subsystem/MF array/MF26 200-207 ==
  In1 : Inport  OutDataType=sfix(16)  OutScaling=2^0
  Add : Sum  Inputs=++++++++  OutDataType=sfix(16)  OutScaling=2^-10
  Subsystem : Subsystem
  Out1 : Outport  OutDataType=sfix(16)  OutScaling=2^0
  wires:
  Add/1 -> Out1/1
  In1/1 -> Subsystem/1(In1)
  Subsystem/1(Out1) -> Add/1
  Subsystem/2(Out5) -> Add/2
  Subsystem/3(Out10) -> Add/3
  Subsystem/4(Out12) -> Add/4
  Subsystem/5(Out13) -> Add/5
  Subsystem/6(Out16) -> Add/6
  Subsystem/7(Out17) -> Add/7
  Subsystem/8(Out18) -> Add/8

== system dsss/PN_DOPPLE/MF Subsystem/MF array/MF27 208-215 ==
  In1 : Inport  OutDataType=sfix(16)  OutScaling=2^0
  Add : Sum  Inputs=++++++++  OutDataType=sfix(16)  OutScaling=2^-10
  Subsystem : Subsystem
  Out1 : Outport  OutDataType=sfix(16)  OutScaling=2^0
  wires:
  Add/1 -> Out1/1
  In1/1 -> Subsystem/1(In1)
  Subsystem/1(Out3) -> Add/1
  Subsystem/2(Out4) -> Add/2
  Subsystem/3(Out7) -> Add/3
  Subsystem/4(Out8) -> Add/4
  Subsystem/5(Out9) -> Add/5
  Subsystem/6(Out11) -> Add/6
  Subsystem/7(Out14) -> Add/7
  Subsystem/8(Out15) -> Add/8

== system dsss/PN_DOPPLE/MF Subsystem/MF array/MF28 216-223 ==
  In1 : Inport  OutDataType=sfix(16)  OutScaling=2^0
  Add : Sum  Inputs=++++++++  OutDataType=sfix(16)  OutScaling=2^-10
  Subsystem : Subsystem
  Out1 : Outport  OutDataType=sfix(16)  OutScaling=2^0
  wires:
  In1/1 -> Subsystem/1(In1)
  Add/1 -> Out1/1
  Subsystem/1(Out1) -> Add/1
  Subsystem/2(Out5) -> Add/2
  Subsystem/3(Out10) -> Add/3
  Subsystem/4(Out12) -> Add/4
  Subsystem/5(Out13) -> Add/5
  Subsystem/6(Out16) -> Add/6
  Subsystem/7(Out17) -> Add/7
  Subsystem/8(Out18) -> Add/8

== system dsss/PN_DOPPLE/MF Subsystem/MF array/MF29 224-231 ==
  In1 : Inport  OutDataType=sfix(16)  OutScaling=2^0
  Add : Sum  Inputs=++++++++  OutDataType=sfix(16)  OutScaling=2^-10
  Subsystem : Subsystem
  Out1 : Outport  OutDataType=sfix(16)  OutScaling=2^0
  wires:
  In1/1 -> Subsystem/1(In1)
  Add/1 -> Out1/1
  Subsystem/1(Out3) -> Add/1
  Subsystem/2(Out4) -> Add/2
  Subsystem/3(Out7) -> Add/3
  Subsystem/4(Out8) -> Add/4
  Subsystem/5(Out9) -> Add/5
  Subsystem/6(Out11) -> Add/6
  Subsystem/7(Out14) -> Add/7
  Subsystem/8(Out15) -> Add/8

== system dsss/PN_DOPPLE/MF Subsystem/MF array/MF3 16-23 ==
  In1 : Inport  OutDataType=sfix(16)  OutScaling=2^0
  Add : Sum  Inputs=++++++++  OutDataType=sfix(16)  OutScaling=2^-10
  Subsystem : Subsystem
  Out1 : Outport  OutDataType=sfix(16)  OutScaling=2^0
  wires:
  In1/1 -> Subsystem/1(In1)
  Add/1 -> Out1/1
  Subsystem/1(Out1) -> Add/1
  Subsystem/2(Out2) -> Add/2
  Subsystem/3(Out3) -> Add/3
  Subsystem/4(Out4) -> Add/4
  Subsystem/5(Out5) -> Add/5
  Subsystem/6(Out6) -> Add/6
  Subsystem/7(Out7) -> Add/7
  Subsystem/8(Out8) -> Add/8

== system dsss/PN_DOPPLE/MF Subsystem/MF array/MF30 232-239 ==
  In1 : Inport  OutDataType=sfix(16)  OutScaling=2^0
  Add : Sum  Inputs=++++++++  OutDataType=sfix(16)  OutScaling=2^-10
  Subsystem : Subsystem
  Out1 : Outport  OutDataType=sfix(16)  OutScaling=2^0
  wires:
  Add/1 -> Out1/1
  In1/1 -> Subsystem/1(In1)
  Subsystem/1(Out1) -> Add/1
  Subsystem/2(Out5) -> Add/2
  Subsystem/3(Out10) -> Add/3
  Subsystem/4(Out12) -> Add/4
  Subsystem/5(Out13) -> Add/5
  Subsystem/6(Out16) -> Add/6
  Subsystem/7(Out17) -> Add/7
  Subsystem/8(Out18) -> Add/8

== system dsss/PN_DOPPLE/MF Subsystem/MF array/MF31 240-247 ==
  In1 : Inport  OutDataType=sfix(16)  OutScaling=2^0
  Add : Sum  Inputs=++++++++  OutDataType=sfix(16)  OutScaling=2^-10
  Subsystem : Subsystem
  Out1 : Outport  OutDataType=sfix(16)  OutScaling=2^0
  wires:
  Add/1 -> Out1/1
  In1/1 -> Subsystem/1(In1)
  Subsystem/1(Out2) -> Add/1
  Subsystem/2(Out3) -> Add/2
  Subsystem/3(Out6) -> Add/3
  Subsystem/4(Out7) -> Add/4
  Subsystem/5(Out9) -> Add/5
  Subsystem/6(Out11) -> Add/6
  Subsystem/7(Out14) -> Add/7
  Subsystem/8(Out15) -> Add/8

== system dsss/PN_DOPPLE/MF Subsystem/MF array/MF32 248-255 ==
  In1 : Inport  OutDataType=sfix(16)  OutScaling=2^0
  Add : Sum  Inputs=++++++++  OutDataType=sfix(16)  OutScaling=2^-10
  Subsystem : Subsystem
  Out1 : Outport  OutDataType=sfix(16)  OutScaling=2^0
  wires:
  In1/1 -> Subsystem/1(In1)
  Add/1 -> Out1/1
  Subsystem/1(Out1) -> Add/1
  Subsystem/2(Out4) -> Add/2
  Subsystem/3(Out5) -> Add/3
  Subsystem/4(Out8) -> Add/4
  Subsystem/5(Out10) -> Add/5
  Subsystem/6(Out12) -> Add/6
  Subsystem/7(Out13) -> Add/7
  Subsystem/8(Out16) -> Add/8

== system dsss/PN_DOPPLE/MF Subsystem/MF array/MF4 24-31 ==
  In1 : Inport  OutDataType=sfix(16)  OutScaling=2^0
  Add : Sum  Inputs=++++++++  OutDataType=sfix(16)  OutScaling=2^-10
  Subsystem : Subsystem
  Out1 : Outport  OutDataType=sfix(16)  OutScaling=2^0
  wires:
  Subsystem/8(Out8) -> Add/8
  Subsystem/7(Out7) -> Add/7
  Subsystem/6(Out6) -> Add/6
  Subsystem/5(Out5) -> Add/5
  Subsystem/4(Out4) -> Add/4
  Subsystem/3(Out3) -> Add/3
  Subsystem/2(Out2) -> Add/2
  Subsystem/1(Out1) -> Add/1
  Add/1 -> Out1/1
  In1/1 -> Subsystem/1(In1)

== system dsss/PN_DOPPLE/MF Subsystem/MF array/MF5 32-39 ==
  In1 : Inport  OutDataType=sfix(16)  OutScaling=2^0
  Add : Sum  Inputs=++++++++  OutDataType=sfix(16)  OutScaling=2^-10
  Subsystem : Subsystem
  Out1 : Outport  OutDataType=sfix(16)  OutScaling=2^0
  wires:
  Add/1 -> Out1/1
  In1/1 -> Subsystem/1(In1)
  Subsystem/1(Out1) -> Add/1
  Subsystem/2(Out2) -> Add/2
  Subsystem/3(Out3) -> Add/3
  Subsystem/4(Out4) -> Add/4
  Subsystem/5(Out5) -> Add/5
  Subsystem/6(Out6) -> Add/6
  Subsystem/7(Out7) -> Add/7
  Subsystem/8(Out8) -> Add/8

== system dsss/PN_DOPPLE/MF Subsystem/MF array/MF6 40-47 ==
  In1 : Inport  OutDataType=sfix(16)  OutScaling=2^0
  Add : Sum  Inputs=++++++++  OutDataType=sfix(16)  OutScaling=2^-10
  Subsystem : Subsystem
  Out1 : Outport  OutDataType=sfix(16)  OutScaling=2^0
  wires:
  Subsystem/8(Out8) -> Add/8
  Subsystem/7(Out7) -> Add/7
  Subsystem/6(Out6) -> Add/6
  Subsystem/5(Out5) -> Add/5
  Subsystem/4(Out4) -> Add/4
  Subsystem/3(Out3) -> Add/3
  Subsystem/2(Out2) -> Add/2
  Subsystem/1(Out1) -> Add/1
  In1/1 -> Subsystem/1(In1)
  Add/1 -> Out1/1

== system dsss/PN_DOPPLE/MF Subsystem/MF array/MF7 48-55 ==
  In1 : Inport  OutDataType=sfix(16)  OutScaling=2^0
  Add : Sum  Inputs=++++++++  OutDataType=sfix(16)  OutScaling=2^-10
  Subsystem : Subsystem
  Out1 : Outport  OutDataType=sfix(16)  OutScaling=2^0
  wires:
  In1/1 -> Subsystem/1(In1)
  Add/1 -> Out1/1
  Subsystem/1(Out1) -> Add/1
  Subsystem/2(Out2) -> Add/2
  Subsystem/3(Out3) -> Add/3
  Subsystem/4(Out4) -> Add/4
  Subsystem/5(Out5) -> Add/5
  Subsystem/6(Out6) -> Add/6
  Subsystem/7(Out7) -> Add/7
  Subsystem/8(Out8) -> Add/8

== system dsss/PN_DOPPLE/MF Subsystem/MF array/MF8 55-62 ==
  In1 : Inport  OutDataType=sfix(16)  OutScaling=2^0
  Add : Sum  Inputs=++++++++  OutDataType=sfix(16)  OutScaling=2^-10
  Subsystem : Subsystem
  Out1 : Outport  OutDataType=sfix(16)  OutScaling=2^0
  wires:
  Subsystem/8(Out8) -> Add/8
  Subsystem/7(Out7) -> Add/7
  Subsystem/6(Out6) -> Add/6
  Subsystem/5(Out5) -> Add/5
  Subsystem/4(Out4) -> Add/4
  Subsystem/3(Out3) -> Add/3
  Subsystem/2(Out2) -> Add/2
  Subsystem/1(Out1) -> Add/1
  Add/1 -> Out1/1
  In1/1 -> Subsystem/1(In1)

== system dsss/PN_DOPPLE/MF Subsystem/MF array/MF9 64-71 ==
  In1 : Inport  OutDataType=sfix(16)  OutScaling=2^0
  Add : Sum  Inputs=++++++++  OutDataType=sfix(16)  OutScaling=2^-10
  Subsystem : Subsystem
  Out1 : Outport  OutDataType=sfix(16)  OutScaling=2^0
  wires:
  Add/1 -> Out1/1
  In1/1 -> Subsystem/1(In1)
  Subsystem/1(Out1) -> Add/1
  Subsystem/2(Out2) -> Add/2
  Subsystem/3(Out3) -> Add/3
  Subsystem/4(Out4) -> Add/4
  Subsystem/5(Out5) -> Add/5
  Subsystem/6(Out6) -> Add/6
  Subsystem/7(Out7) -> Add/7
  Subsystem/8(Out8) -> Add/8

== system dsss/PN_DOPPLE/Local PN/local PN sequence Include Track/Local System/[1 0 0 1 1 1 0 1]PN ==
  note: 1 0 0 0 1 1 1 0 1
  In1 : Inport  OutDataType=sfix(16)  OutScaling=2^0
  Trigger : TriggerPort
  Enabled Subsystem : Subsystem  TreatAsAtomicUnit=on
  Enabled Subsystem1 : Subsystem  TreatAsAtomicUnit=on
  Enabled Subsystem2 : Subsystem  TreatAsAtomicUnit=on
  Enabled Subsystem3 : Subsystem  TreatAsAtomicUnit=on
  Enabled Subsystem4 : Subsystem  TreatAsAtomicUnit=on
  Enabled Subsystem5 : Subsystem  TreatAsAtomicUnit=on
  Enabled Subsystem6 : Subsystem  TreatAsAtomicUnit=on
  Enabled Subsystem7 : Subsystem  TreatAsAtomicUnit=on
  Logical Operator : Logic  Operator=XOR  Inputs=4  AllPortsSameDT=off  OutDataTypeMode=boolean  OutDataTypeStr=boolean
  Out1 : Outport  OutDataType=sfix(16)  OutScaling=2^0
  wires:
  Enabled Subsystem/1(Out1) -> Enabled Subsystem3/1(In1)
  Enabled Subsystem3/1(Out1) -> Enabled Subsystem4/1(In1)
  In1/1 -> Enabled Subsystem/Enable, Enabled Subsystem4/Enable, Enabled Subsystem1/Enable, Enabled Subsystem2/Enable, Enabled Subsystem5/Enable, Enabled Subsystem6/Enable, Enabled Subsystem7/Enable, Enabled Subsystem3/Enable
  Logical Operator/1 -> Enabled Subsystem/1(In1)
  Enabled Subsystem7/1(Out1) -> Logical Operator/1, Out1/1
  Enabled Subsystem4/1(Out1) -> Enabled Subsystem1/1(In1)
  Enabled Subsystem6/1(Out1) -> Enabled Subsystem7/1(In1)
  Enabled Subsystem1/1(Out1) -> Enabled Subsystem2/1(In1), Logical Operator/4
  Enabled Subsystem2/1(Out1) -> Enabled Subsystem5/1(In1), Logical Operator/3
  Enabled Subsystem5/1(Out1) -> Enabled Subsystem6/1(In1), Logical Operator/2

== system dsss/PN_DOPPLE/MF Subsystem/MF array/MF1 0-7/Subsystem ==
  In1 : Inport  OutDataType=sfix(16)  OutScaling=2^0
  Constant1 : Constant  OutDataType=sfix(16)  OutScaling=2^0
  Constant{2..3,5..7} (5 alike) : Constant  Value=-1  OutDataType=sfix(16)  OutScaling=2^0
  Constant4 : Constant  OutDataType=sfix(16)  OutScaling=2^0
  Constant8 : Constant  OutDataType=sfix(16)  OutScaling=2^0
  Integer Delay1 : simulink/Discrete/Integer Delay  vinit=0.0  samptime=-1  NumDelays=3
  Integer Delay2 : simulink/Discrete/Integer Delay  vinit=0.0  samptime=-1  NumDelays=2
  Integer Delay3 : simulink/Discrete/Integer Delay  vinit=0.0  samptime=-1  NumDelays=1
  Integer Delay5 : simulink/Discrete/Integer Delay  vinit=0.0  samptime=-1  NumDelays=7
  Integer Delay6 : simulink/Discrete/Integer Delay  vinit=0.0  samptime=-1  NumDelays=6
  Integer Delay7 : simulink/Discrete/Integer Delay  vinit=0.0  samptime=-1  NumDelays=5
  Integer Delay8 : simulink/Discrete/Integer Delay  vinit=0.0  samptime=-1  NumDelays=4
  Product{1..8} (8 alike) : Product  OutDataType=sfix(16)  OutScaling=2^0  RndMeth=Zero
  Out1 : Outport  OutDataType=sfix(16)  OutScaling=2^0
  Out2 : Outport  Port=2  OutDataType=sfix(16)  OutScaling=2^0
  Out3 : Outport  Port=3  OutDataType=sfix(16)  OutScaling=2^0
  Out4 : Outport  Port=4  OutDataType=sfix(16)  OutScaling=2^0
  Out5 : Outport  Port=5  OutDataType=sfix(16)  OutScaling=2^0
  Out6 : Outport  Port=6  OutDataType=sfix(16)  OutScaling=2^0
  Out7 : Outport  Port=7  OutDataType=sfix(16)  OutScaling=2^0
  Out8 : Outport  Port=8  OutDataType=sfix(16)  OutScaling=2^0
  wires:
  Product6/1 -> Out8/1
  Product2/1 -> Out4/1
  Product5/1 -> Out7/1
  Product1/1 -> Out3/1
  Product8/1 -> Out6/1
  Product4/1 -> Out2/1
  Product7/1 -> Out5/1
  Product3/1 -> Out1/1
  Integer Delay8/1 -> Product7/1
  Constant6/1 -> Product7/2
  Integer Delay7/1 -> Product8/1
  Constant7/1 -> Product8/2
  Integer Delay6/1 -> Product5/1
  Constant5/1 -> Product5/2
  Integer Delay5/1 -> Product6/1
  Constant8/1 -> Product6/2
  Constant2/1 -> Product3/2
  Integer Delay3/1 -> Product4/1
  Constant3/1 -> Product4/2
  Integer Delay2/1 -> Product1/1
  Constant1/1 -> Product1/2
  Integer Delay1/1 -> Product2/1
  Constant4/1 -> Product2/2
  In1/1 -> Product3/1, Integer Delay1/1, Integer Delay2/1, Integer Delay3/1, Integer Delay8/1, Integer Delay7/1, Integer Delay6/1, Integer Delay5/1

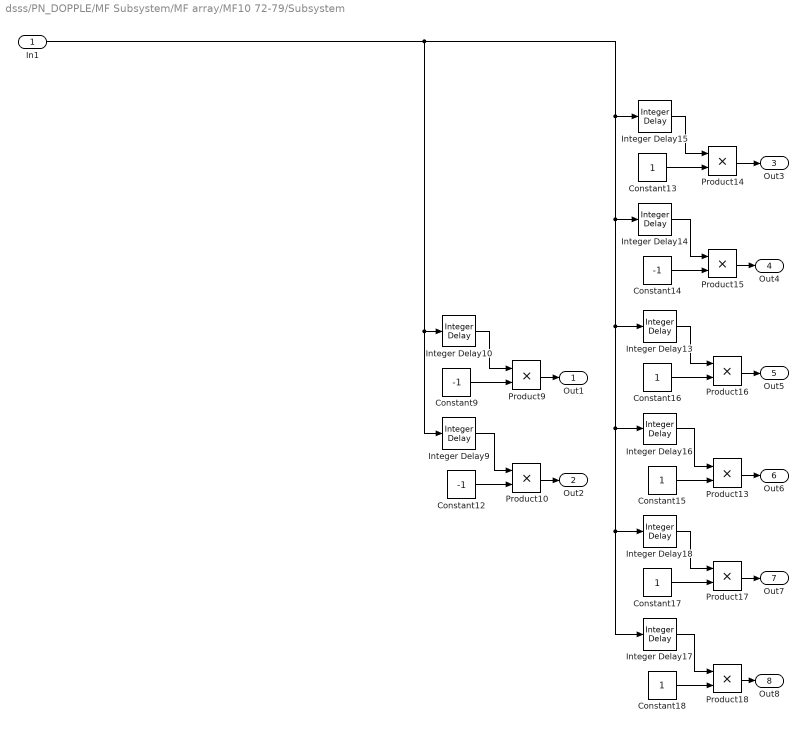
== system dsss/PN_DOPPLE/MF Subsystem/MF array/MF10 72-79/Subsystem ==
  In1 : Inport  OutDataType=sfix(16)  OutScaling=2^0
  Constant12 : Constant  Value=-1  OutDataType=sfix(16)  OutScaling=2^0
  Constant{13,15..18} (5 alike) : Constant  OutDataType=sfix(16)  OutScaling=2^0
  Constant14 : Constant  Value=-1  OutDataType=sfix(16)  OutScaling=2^0
  Constant9 : Constant  Value=-1  OutDataType=sfix(16)  OutScaling=2^0
  Integer Delay10 : simulink/Discrete/Integer Delay  vinit=0.0  samptime=-1  NumDelays=72
  Integer Delay13 : simulink/Discrete/Integer Delay  vinit=0.0  samptime=-1  NumDelays=76
  Integer Delay14 : simulink/Discrete/Integer Delay  vinit=0.0  samptime=-1  NumDelays=75
  Integer Delay15 : simulink/Discrete/Integer Delay  vinit=0.0  samptime=-1  NumDelays=74
  Integer Delay16 : simulink/Discrete/Integer Delay  vinit=0.0  samptime=-1  NumDelays=77
  Integer Delay17 : simulink/Discrete/Integer Delay  vinit=0.0  samptime=-1  NumDelays=79
  Integer Delay18 : simulink/Discrete/Integer Delay  vinit=0.0  samptime=-1  NumDelays=78
  Integer Delay9 : simulink/Discrete/Integer Delay  vinit=0.0  samptime=-1  NumDelays=73
  Product{9..10,13..18} (8 alike) : Product  OutDataType=sfix(16)  OutScaling=2^0  RndMeth=Zero
  Out1 : Outport  OutDataType=sfix(16)  OutScaling=2^0
  Out2 : Outport  Port=2  OutDataType=sfix(16)  OutScaling=2^0
  Out3 : Outport  Port=3  OutDataType=sfix(16)  OutScaling=2^0
  Out4 : Outport  Port=4  OutDataType=sfix(16)  OutScaling=2^0
  Out5 : Outport  Port=5  OutDataType=sfix(16)  OutScaling=2^0
  Out6 : Outport  Port=6  OutDataType=sfix(16)  OutScaling=2^0
  Out7 : Outport  Port=7  OutDataType=sfix(16)  OutScaling=2^0
  Out8 : Outport  Port=8  OutDataType=sfix(16)  OutScaling=2^0
  wires:
  In1/1 -> Integer Delay13/1, Integer Delay16/1, Integer Delay18/1, Integer Delay17/1, Integer Delay14/1, Integer Delay15/1, Integer Delay9/1, Integer Delay10/1
  Integer Delay9/1 -> Product10/1
  Constant9/1 -> Product9/2
  Integer Delay10/1 -> Product9/1
  Integer Delay16/1 -> Product13/1
  Constant16/1 -> Product16/2
  Integer Delay13/1 -> Product16/1
  Constant14/1 -> Product15/2
  Integer Delay14/1 -> Product15/1
  Constant13/1 -> Product14/2
  Integer Delay15/1 -> Product14/1
  Constant12/1 -> Product10/2
  Constant15/1 -> Product13/2
  Product15/1 -> Out4/1
  Product16/1 -> Out5/1
  Product9/1 -> Out1/1
  Product13/1 -> Out6/1
  Product10/1 -> Out2/1
  Product18/1 -> Out8/1
  Product17/1 -> Out7/1
  Constant17/1 -> Product17/2
  Integer Delay17/1 -> Product18/1
  Constant18/1 -> Product18/2
  Integer Delay18/1 -> Product17/1
  Product14/1 -> Out3/1

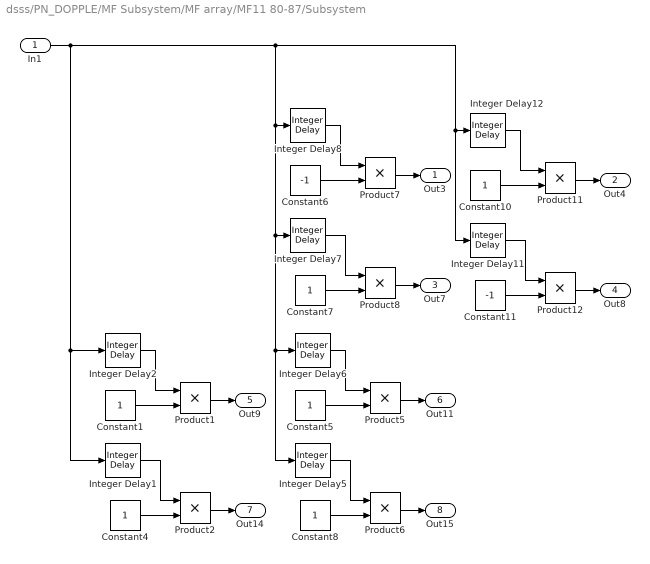
== system dsss/PN_DOPPLE/MF Subsystem/MF array/MF11 80-87/Subsystem ==
  In1 : Inport  OutDataType=sfix(16)  OutScaling=2^0
  Constant{1,4..5,7..8,10} (6 alike) : Constant  OutDataType=sfix(16)  OutScaling=2^0
  Constant11 : Constant  Value=-1  OutDataType=sfix(16)  OutScaling=2^0
  Constant6 : Constant  Value=-1  OutDataType=sfix(16)  OutScaling=2^0
  Integer Delay1 : simulink/Discrete/Integer Delay  vinit=0.0  samptime=-1  NumDelays=81
  Integer Delay11 : simulink/Discrete/Integer Delay  vinit=0.0  samptime=-1  NumDelays=87
  Integer Delay12 : simulink/Discrete/Integer Delay  vinit=0.0  samptime=-1  NumDelays=86
  Integer Delay2 : simulink/Discrete/Integer Delay  vinit=0.0  samptime=-1  NumDelays=80
  Integer Delay5 : simulink/Discrete/Integer Delay  vinit=0.0  samptime=-1  NumDelays=85
  Integer Delay6 : simulink/Discrete/Integer Delay  vinit=0.0  samptime=-1  NumDelays=84
  Integer Delay7 : simulink/Discrete/Integer Delay  vinit=0.0  samptime=-1  NumDelays=83
  Integer Delay8 : simulink/Discrete/Integer Delay  vinit=0.0  samptime=-1  NumDelays=82
  Product{1..2,5..8,11..12} (8 alike) : Product  OutDataType=sfix(16)  OutScaling=2^0  RndMeth=Zero
  Out3 : Outport  OutDataType=sfix(16)  OutScaling=2^0
  Out4 : Outport  Port=2  OutDataType=sfix(16)  OutScaling=2^0
  Out7 : Outport  Port=3  OutDataType=sfix(16)  OutScaling=2^0
  Out8 : Outport  Port=4  OutDataType=sfix(16)  OutScaling=2^0
  Out9 : Outport  Port=5  OutDataType=sfix(16)  OutScaling=2^0
  Out11 : Outport  Port=6  OutDataType=sfix(16)  OutScaling=2^0
  Out14 : Outport  Port=7  OutDataType=sfix(16)  OutScaling=2^0
  Out15 : Outport  Port=8  OutDataType=sfix(16)  OutScaling=2^0
  wires:
  In1/1 -> Integer Delay2/1, Integer Delay1/1, Integer Delay5/1, Integer Delay6/1, Integer Delay7/1, Integer Delay8/1, Integer Delay12/1, Integer Delay11/1
  Constant4/1 -> Product2/2
  Integer Delay1/1 -> Product2/1
  Constant1/1 -> Product1/2
  Integer Delay2/1 -> Product1/1
  Constant8/1 -> Product6/2
  Integer Delay5/1 -> Product6/1
  Constant5/1 -> Product5/2
  Integer Delay6/1 -> Product5/1
  Constant7/1 -> Product8/2
  Integer Delay7/1 -> Product8/1
  Constant6/1 -> Product7/2
  Integer Delay8/1 -> Product7/1
  Constant11/1 -> Product12/2
  Integer Delay11/1 -> Product12/1
  Constant10/1 -> Product11/2
  Integer Delay12/1 -> Product11/1
  Product7/1 -> Out3/1
  Product11/1 -> Out4/1
  Product8/1 -> Out7/1
  Product12/1 -> Out8/1
  Product1/1 -> Out9/1
  Product5/1 -> Out11/1
  Product2/1 -> Out14/1
  Product6/1 -> Out15/1

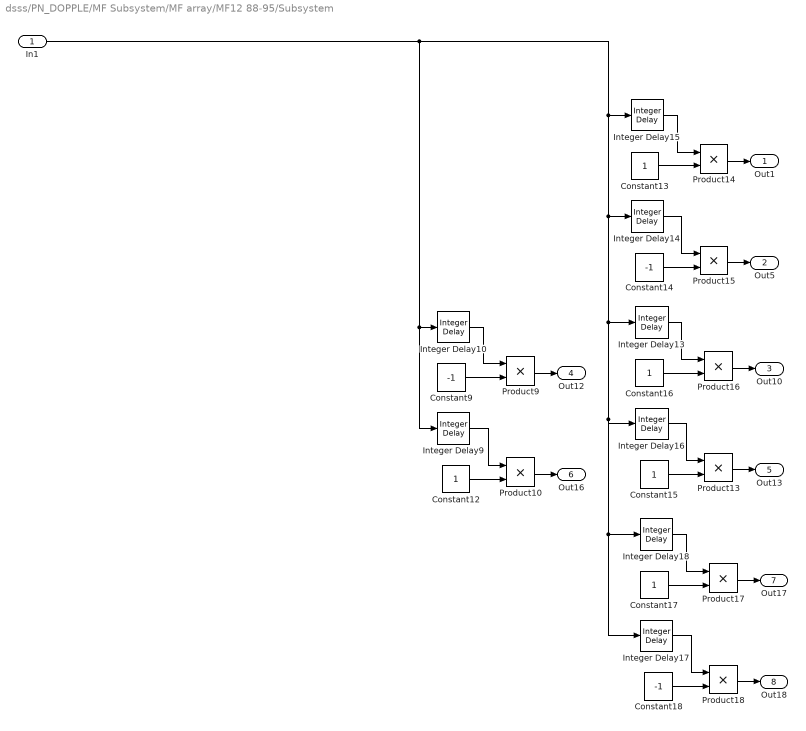
== system dsss/PN_DOPPLE/MF Subsystem/MF array/MF12 88-95/Subsystem ==
  In1 : Inport  OutDataType=sfix(16)  OutScaling=2^0
  Constant{12..13,15..17} (5 alike) : Constant  OutDataType=sfix(16)  OutScaling=2^0
  Constant14 : Constant  Value=-1  OutDataType=sfix(16)  OutScaling=2^0
  Constant18 : Constant  Value=-1  OutDataType=sfix(16)  OutScaling=2^0
  Constant9 : Constant  Value=-1  OutDataType=sfix(16)  OutScaling=2^0
  Integer Delay10 : simulink/Discrete/Integer Delay  vinit=0.0  samptime=-1  NumDelays=88
  Integer Delay13 : simulink/Discrete/Integer Delay  vinit=0.0  samptime=-1  NumDelays=92
  Integer Delay14 : simulink/Discrete/Integer Delay  vinit=0.0  samptime=-1  NumDelays=91
  Integer Delay15 : simulink/Discrete/Integer Delay  vinit=0.0  samptime=-1  NumDelays=90
  Integer Delay16 : simulink/Discrete/Integer Delay  vinit=0.0  samptime=-1  NumDelays=93
  Integer Delay17 : simulink/Discrete/Integer Delay  vinit=0  samptime=-1  NumDelays=95
  Integer Delay18 : simulink/Discrete/Integer Delay  vinit=0  samptime=-1  NumDelays=94
  Integer Delay9 : simulink/Discrete/Integer Delay  vinit=0.0  samptime=-1  NumDelays=89
  Product{9..10,13..18} (8 alike) : Product  OutDataType=sfix(16)  OutScaling=2^0  RndMeth=Zero
  Out1 : Outport  OutDataType=sfix(16)  OutScaling=2^0
  Out5 : Outport  Port=2  OutDataType=sfix(16)  OutScaling=2^0
  Out10 : Outport  Port=3  OutDataType=sfix(16)  OutScaling=2^0
  Out12 : Outport  Port=4  OutDataType=sfix(16)  OutScaling=2^0
  Out13 : Outport  Port=5  OutDataType=sfix(16)  OutScaling=2^0
  Out16 : Outport  Port=6  OutDataType=sfix(16)  OutScaling=2^0
  Out17 : Outport  Port=7  OutDataType=sfix(16)  OutScaling=2^0
  Out18 : Outport  Port=8  OutDataType=sfix(16)  OutScaling=2^0
  wires:
  Product10/1 -> Out16/1
  Product13/1 -> Out13/1
  Product9/1 -> Out12/1
  Product16/1 -> Out10/1
  Product15/1 -> Out5/1
  Product14/1 -> Out1/1
  Constant15/1 -> Product13/2
  Constant12/1 -> Product10/2
  Integer Delay15/1 -> Product14/1
  Constant13/1 -> Product14/2
  Integer Delay14/1 -> Product15/1
  Constant14/1 -> Product15/2
  Integer Delay13/1 -> Product16/1
  Constant16/1 -> Product16/2
  Integer Delay16/1 -> Product13/1
  Integer Delay10/1 -> Product9/1
  Constant9/1 -> Product9/2
  Integer Delay9/1 -> Product10/1
  In1/1 -> Integer Delay15/1, Integer Delay14/1, Integer Delay13/1, Integer Delay16/1, Integer Delay18/1, Integer Delay17/1, Integer Delay10/1, Integer Delay9/1
  Constant18/1 -> Product18/2
  Integer Delay17/1 -> Product18/1
  Constant17/1 -> Product17/2
  Product17/1 -> Out17/1
  Product18/1 -> Out18/1
  Integer Delay18/1 -> Product17/1
